simulink model "CKF_LQRCombined"  (R2014b)
settings: Solver=ode4  StartTime=0.0  StopTime=20  FixedStep=0.01  RelTol=1e-3
values from neighbouring files (symbols this model uses):
  A = [0 0 1 0 ... (first row only)    [InitialzeWorkspace.m]
  Bu = [0 ... (first row only)    [InitialzeWorkspace.m]
  Bw = [0.5 ... (first row only)    [InitialzeWorkspace.m]
  C = [1 0 0 0]    [InitialzeWorkspace.m]
  Se_init = zeros(4,4)    [InitialzeWorkspace.m]
  Sv = 0.005    [InitialzeWorkspace.m]
  Sw = 0.002^2    (= 4e-06)    [InitialzeWorkspace.m]
  X_init = [0 0 0 0]    [InitialzeWorkspace.m]
undefined symbols (not defined in the file or in its folder): K_LQR
settings Model: Creator=E38497  LastModifiedBy=Pranav
settings DebuggingCC: UnderspecifiedInitializationDetection=Classic  MergeDetectMultiDrivingBlocksExec=none

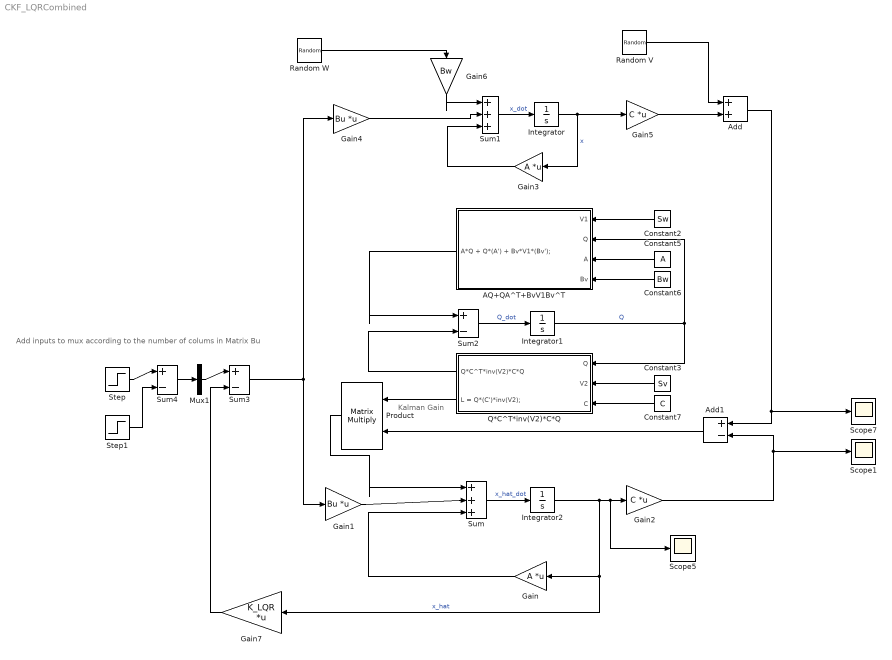
== system CKF_LQRCombined ==
  note: Kalman Gain
  note: Add inputs to mux according to the number of colums in Matrix Bu
  AQ+QA^T+BvV1Bv^T : Subsystem  TreatAsAtomicUnit=on
  Add : Sum
  Add1 : Sum  Inputs=+-
  Constant2 : Constant  Value=Sw
  Constant3 : Constant  Value=Sv
  Constant5 : Constant  Value=A  VectorParams1D=off
  Constant6 : Constant  Value=Bw  VectorParams1D=off
  Constant7 : Constant  Value=C  VectorParams1D=off
  Gain : Gain  Gain=A  Multiplication=Matrix(K*u)
  Gain1 : Gain  Gain=Bu  Multiplication=Matrix(K*u)
  Gain2 : Gain  Gain=C  Multiplication=Matrix(K*u)
  Gain3 : Gain  Gain=A  Multiplication=Matrix(K*u)
  Gain4 : Gain  Gain=Bu  Multiplication=Matrix(K*u)
  Gain5 : Gain  Gain=C  Multiplication=Matrix(K*u)
  Gain6 : Gain  Gain=Bw
  Gain7 : Gain  Gain=K_LQR  Multiplication=Matrix(K*u)
  Integrator : Integrator  InitialCondition=X_init  UpperSaturationLimit=1  LowerSaturationLimit=-1
  Integrator1 : Integrator  InitialCondition=Se_init
  Integrator2 : Integrator  InitialCondition=X_init
  Mux1 : Mux  Inputs=1
  Product : Product  Multiplication=Matrix(*)
  Q*C^T*inv(V2)*C*Q : Subsystem  TreatAsAtomicUnit=on
  Random V : RandomNumber  Variance=Sv
  Random W : RandomNumber  Variance=Sw*2
  Scope1 : Scope
      settings: YMin=-10  YMax=10
  Scope5 : Scope
      settings: YMin=-10  YMax=10  SaveName=ScopeData5
  Scope7 : Scope
      settings: YMin=-10  YMax=10  SaveName=ScopeData7
  Step : Step  After=5  SampleTime=0
  Step1 : Step  Time=1.2  After=0  SampleTime=0
  Sum : Sum  Inputs=|+++
  Sum1 : Sum  Inputs=|+++
  Sum2 : Sum  Inputs=|+-
  Sum3 : Sum  Inputs=|+-
  Sum4 : Sum  Inputs=|+-
  wires:
  Gain/1 -> Sum/3
  Sum/1 -> Integrator2/1  "x_hat_dot"
  Integrator2/1 -> Scope5/1, Gain2/1, Gain/1, Gain7/1  "x_hat"
  Gain4/1 -> Sum1/2
  Gain3/1 -> Sum1/3
  Sum1/1 -> Integrator/1  "x_dot"
  Integrator/1 -> Gain3/1, Gain5/1  "x"
  Gain6/1 -> Sum1/1
  Random V/1 -> Add/1
  Gain2/1 -> Scope1/1, Add1/2
  Integrator1/1 -> Q*C^T*inv(V2)*C*Q/1(Q), AQ+QA^T+BvV1Bv^T/2(Q)  "Q"
  Constant2/1 -> AQ+QA^T+BvV1Bv^T/1(V1)
  AQ+QA^T+BvV1Bv^T/1(A*Q + Q*(A') + Bv*V1*(Bv');) -> Sum2/1
  Q*C^T*inv(V2)*C*Q/1(Q*C^T*inv(V2)*C*Q) -> Sum2/2
  Sum2/1 -> Integrator1/1  "Q_dot"
  Constant3/1 -> Q*C^T*inv(V2)*C*Q/2(V2)
  Q*C^T*inv(V2)*C*Q/2(L = Q*(C')*inv(V2);) -> Product/1
  Constant5/1 -> AQ+QA^T+BvV1Bv^T/3(A)
  Constant6/1 -> AQ+QA^T+BvV1Bv^T/4(Bv)
  Constant7/1 -> Q*C^T*inv(V2)*C*Q/3(C)
  Gain1/1 -> Sum/2
  Product/1 -> Sum/1
  Add1/1 -> Product/2
  Random W/1 -> Gain6/1
  Gain7/1 -> Sum3/2
  Gain5/1 -> Add/2
  Step/1 -> Sum4/1
  Step1/1 -> Sum4/2
  Sum3/1 -> Gain1/1, Gain4/1
  Sum4/1 -> Mux1/1
  Add/1 -> Scope7/1, Add1/1
  Mux1/1 -> Sum3/1

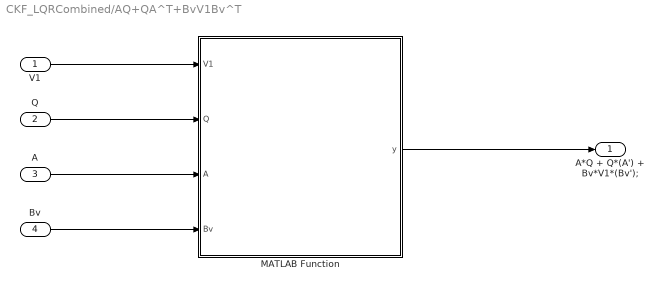
== system CKF_LQRCombined/AQ+QA^T+BvV1Bv^T ==
  V1 : Inport
  Q : Inport  Port=2
  A : Inport  Port=3
  Bv : Inport  Port=4
  MATLAB Function : MATLAB Function  TreatAsAtomicUnit=on
  A*Q + Q*(A') + Bv*V1*(Bv'); : Outport
  wires:
  V1/1 -> MATLAB Function/1(V1)
  MATLAB Function/1(y) -> A*Q + Q*(A') + Bv*V1*(Bv');/1
  Q/1 -> MATLAB Function/2(Q)
  A/1 -> MATLAB Function/3(A)
  Bv/1 -> MATLAB Function/4(Bv)

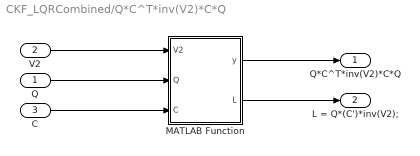
== system CKF_LQRCombined/Q*C^T*inv(V2)*C*Q ==
  Q : Inport
  V2 : Inport  Port=2
  C : Inport  Port=3
  MATLAB Function : MATLAB Function  TreatAsAtomicUnit=on
  Q*C^T*inv(V2)*C*Q : Outport
  L = Q*(C')*inv(V2); : Outport  Port=2
  wires:
  V2/1 -> MATLAB Function/1(V2)
  MATLAB Function/1(y) -> Q*C^T*inv(V2)*C*Q/1
  Q/1 -> MATLAB Function/2(Q)
  C/1 -> MATLAB Function/3(C)
  MATLAB Function/2(L) -> L = Q*(C')*inv(V2);/1

== matlab function CKF_LQRCombined/Q*C^T*inv(V2)*C*Q/MATLAB Function ==
  data: V2 input; y output; Q input; L output; C input
function [y,L] = fcn(V2,Q,C)
y = Q*C'*((V2)\C)*Q;
L = Q*C'/(V2);

% y = Q*C'*inv(V2)*C*Q;
% L = Q*C'*inv(V2);

== matlab function CKF_LQRCombined/AQ+QA^T+BvV1Bv^T/MATLAB Function ==
  data: V1 input; y output; Q input; A input; Bv input
function y = fcn(V1,Q,A,Bv)
%#codegen
% AQ+QA^T+BvV1Bv^T
y = A*Q + Q*(A') + Bv*V1*(Bv');
